simulink model "roll_simulink"  (R2018b)
settings: Solver=VariableStepAuto  StartTime=0.0  StopTime=10.0  RelTol=1e-3
values from neighbouring files (symbols this model uses):
  beta = 63.4*pi/180    (= 1.10653874576)    [Spacecraft.m]
  int_resist = 6    [Spacecraft.m]
  Iw = max([Iw_roll Iw_pitch Iw_yaw])    [Spacecraft.m]    (also in maneuver.m = z2(end)*Is/(4*Omega_max*cos(beta)))
  Ixx = 6000    [Spacecraft.m]
  N = 60    [Spacecraft.m]
  roll_change_angle = 90*pi/180    (= 1.57079632679)    [Spacecraft.m]
libraries: cstblocks x2
settings Model: Creator=Lucie  LastModifiedBy=Lucie

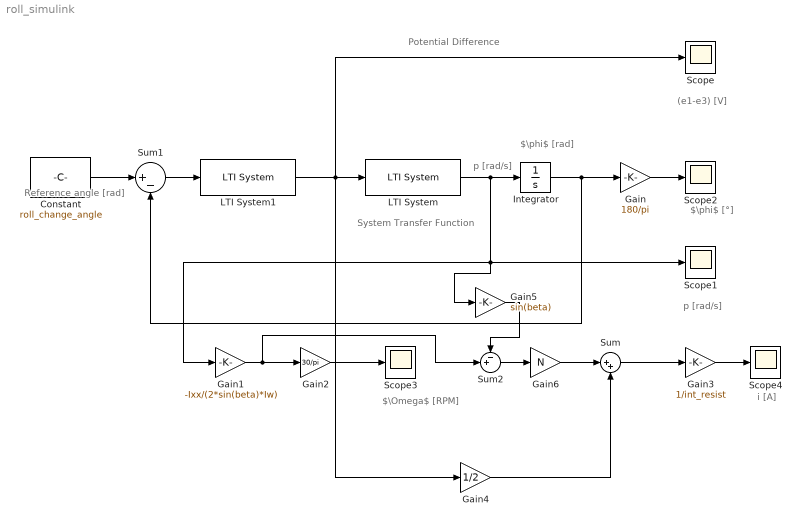
== system roll_simulink ==
  note: System Transfer Function
  note: i [A]
  note: $\Omega$ [RPM]
  note: (e1-e3) [V]
  note: Potential Difference
  note: $\phi$ [rad]
  note: p [rad/s]
  note: Reference angle
      |          [rad]
  note: p [rad/s]
  note: $\phi$ [°]
  Constant : Constant  Value=roll_change_angle
  Gain : Gain  Gain=180/pi
  Gain1 : Gain  Gain=-Ixx/(2*sin(beta)*Iw)
  Gain2 : Gain  Gain=30/pi
  Gain3 : Gain  Gain=1/int_resist
  Gain4 : Gain  Gain=1/2
  Gain5 : Gain  Gain=sin(beta)
  Gain6 : Gain  Gain=N
  Integrator : Integrator
  LTI System : cstblocks/LTI System  sys=Hr  IC=[]
  LTI System1 : cstblocks/LTI System  sys=C  IC=[]
  Scope{,1..4} (5 alike) : Scope
  Sum : Sum  Inputs=|++
  Sum1 : Sum  Inputs=|+-
  Sum2 : Sum  Inputs=-+|
  wires:
  Sum1/1 -> LTI System1/1
  LTI System1/1 -> LTI System/1, Scope/1, Gain4/1
  Constant/1 -> Sum1/1
  Integrator/1 -> Sum1/2, Gain/1
  Gain/1 -> Scope2/1
  Gain1/1 -> Sum2/2, Gain2/1
  Gain2/1 -> Scope3/1
  LTI System/1 -> Gain5/1, Gain1/1, Scope1/1, Integrator/1
  Gain3/1 -> Scope4/1
  Gain5/1 -> Sum2/1
  Sum2/1 -> Gain6/1
  Sum/1 -> Gain3/1
  Gain6/1 -> Sum/1
  Gain4/1 -> Sum/2
